simulink model "Variable_Size_Signal"  (R2019b)
settings: Solver=VariableStepAuto  StartTime=0.0  StopTime=20  RelTol=1e-3
libraries: ModelComposer x1
settings Model: Creator=abehbood  LastModifiedBy=abehbood

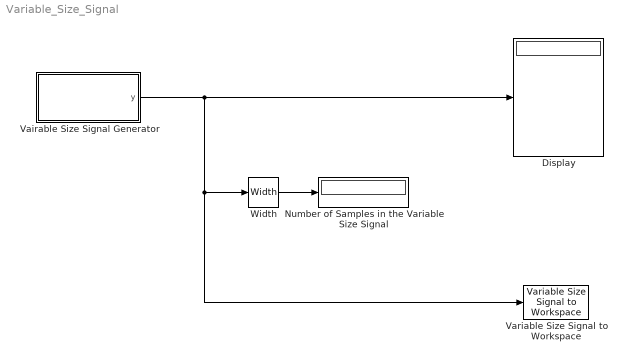
== system Variable_Size_Signal ==
  Display : Display
  Number of Samples in the Variable Size Signal : Display
  Vairable Size Signal Generator : MATLAB Function  TreatAsAtomicUnit=on  SystemSampleTime=1  mask{maxSizeOfVariableSizeSignal=4, outType=Random}
      mask prompts: maxSizeOfVariableSizeSignal "Max Size of Variabel Size Signal"; outType "Number of elements in the output"
      mask help: This block generates a variable size signal output. The number of samples in the output can be random or fixed and are consecutive integer numbers starting from zero.
  Variable Size Signal to Workspace : ModelComposer/Variable Size Signal to Workspace  VariableNameMask=simout
  Width : Width
  wires:
  Vairable Size Signal Generator/1(y) -> Variable Size Signal to Workspace/1, Width/1, Display/1
  Width/1 -> Number of Samples in the Variable Size Signal/1

== matlab function Variable_Size_Signal/Vairable Size Signal Generator ==
  data: y output size=maxSizeOfVariableSizeSignal; maxSizeOfVariableSizeSignal parameter; outType parameter
function y = fcn(maxSizeOfVariableSizeSignal,outType)
%#codegen

persistent out;

if isempty(out)
    out = 0;
    rng(5)
end

if outType == 1
    numOfSamples = randi([0 maxSizeOfVariableSizeSignal],1,1);
else
    numOfSamples = maxSizeOfVariableSizeSignal;
end

y = (out:out+numOfSamples-1)';

out = out + numOfSamples;
